simulink model "mseLoop"  (R2024b)
settings: Solver=VariableStepAuto  StartTime=0.0  StopTime=10.0  RelTol=1e-3
settings Model: Creator=DarianMuresan  LastModifiedBy=ferbe
settings RTWCC: GPUComputeCapability=3.5

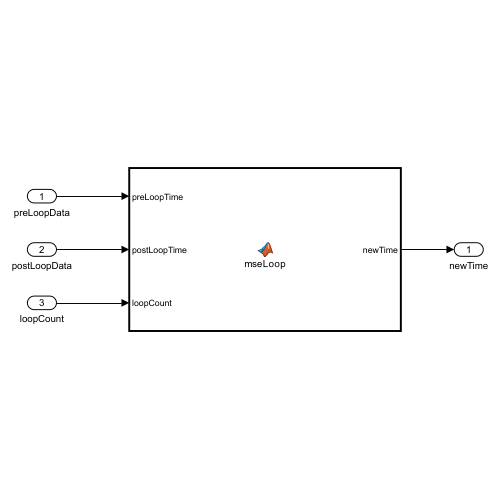
[thumbnail: Simulink's stored preview of the top-level diagram]
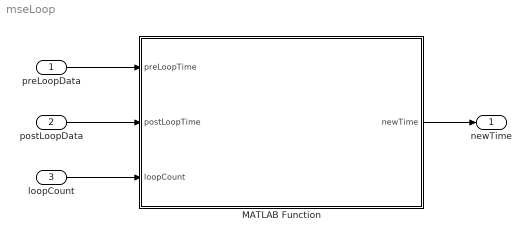
== system mseLoop ==
  preLoopData : Inport
  postLoopData : Inport  Port=2
  loopCount : Inport  Port=3
  MATLAB Function : MATLAB Function  TreatAsAtomicUnit=on
  newTime : Outport
  wires:
  preLoopData/1 -> MATLAB Function/1(preLoopTime)
  postLoopData/1 -> MATLAB Function/2(postLoopTime)
  MATLAB Function/1(newTime) -> newTime/1
  loopCount/1 -> MATLAB Function/3(loopCount)

== matlab function mseLoop/MATLAB Function ==
  data: preLoopTime input; newTime output; postLoopTime input; loopCount input
function newTime = mseLoop(preLoopTime,postLoopTime,loopCount)

% Function to count time generated by loops, assuming each module
% time has been estimated already.
%
% Written by: Darian Muresan
% Modified last: October 12, 2023

newTime = preLoopTime+loopCount*(postLoopTime-preLoopTime);
